simulink model "sampleModel1681_sub"  (R2023a)
settings: Solver=VariableStepAuto  StartTime=0.0  StopTime=10.0  RelTol=1e-3
libraries: hdlsllib x4, simulink x2
settings Model: Creator=user1  LastModifiedBy=user1

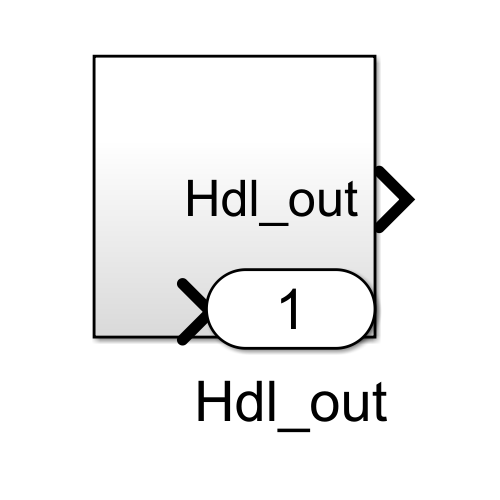
[thumbnail: Simulink's stored preview of the top-level diagram]
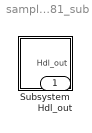
== system sampleModel1681_sub ==
  Subsystem : Subsystem
  Hdl_out : Outport  OutDataTypeStr=uint8

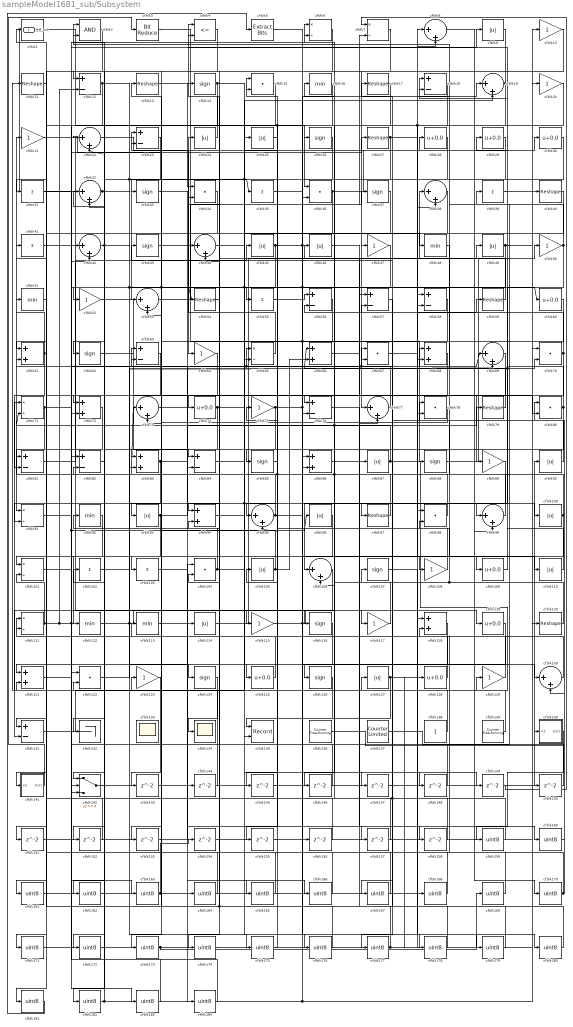
== system sampleModel1681_sub/Subsystem ==
  cfblk1 : simulink/Logic and Bit Operations/Bit Set  iBit=0
      settings: LibrarySourceBlock=|
      | hdlsllib/Logic and Bit
      | Operations/Bit Set
  cfblk{10,20..21,47,50,52,64,75,89,108,115,117,123,129} (14 alike) : Gain  OutDataTypeStr=uint8
  cfblk{9,24..25,45..46,49,87,90,93,96,100,105,110,114,127} (15 alike) : Abs  OutDataTypeStr=uint8  SaturateOnIntegerOverflow=off
  cfblk{6..7,65,71,91,101,111} (7 alike) : Product  Inputs=*/  OutDataTypeStr=uint8  RndMeth=Zero  SaturateOnIntegerOverflow=on
  cfblk{31,35,39,41,55,102..103} (7 alike) : Sum  Inputs=+  OutDataTypeStr=uint8
  cfblk{15,34,36,67,70,78,80,98,104,122} (10 alike) : DotProduct  OutDataTypeStr=uint8
  cfblk{8,19,22,32,38,42,44,53,69,73,77,95,99,106,130} (15 alike) : Sum  Inputs=|++  OutDataTypeStr=uint8
  cfblk{14,26,33,37,43,62,85,88,107,116,124,126} (12 alike) : Signum
  cfblk{28..30,60,74,109,119,125,128} (9 alike) : Bias  Bias=0.0  SaturateOnIntegerOverflow=off
  cfblk{11,13,17,27,40,54,59,79,97,120} (10 alike) : Reshape
  cfblk{16,48,51,92,112..113} (6 alike) : MinMax  OutDataTypeStr=uint8
  cfblk{61,66,68,72,83,86,94,118,121} (9 alike) : Sum  OutDataTypeStr=uint8
  cfblk{12,18,23,56..58,63,76,81..82,84,131} (12 alike) : Sum  Inputs=+-  OutDataTypeStr=uint8
  cfblk132 : Terminator
  cfblk133 : Scope
      settings: Floating=on
  cfblk134 : Scope
  cfblk135 : Record  FileSettingsInternal="{\"entries\":[{\"content\":{\"excelSettings\":{\"content\":{},\"type\":\"Streamout.ExcelSettings\"}},\"type\":\"Streamout.FileSettingStorage\",\"uuid\":\"\"}],\"packageUris\":[\"http:\\/\\/schema.mathworks.com\\/mf0\\/streamout_blocks\\/R2020a\"],\"version\":\"1.0\"}"  Layout=[1 1]  SignalsInternal="{\"entries\":[{\"content\":{\"signals\":[{\"content\":{\"blockPath\":[],\"dimensions\":[1],\"domain\":\"\",\"lineColor\":\"#a2142f\",\"plots\":[1],\"port\":1,\"signalID\":34646,\"signalName\":\"cfblk126\"},\"type\":\"RecordBlkView.Signal\",\"uuid\":\"\"},{\"content\":{\"blockPath\":[],\"dimensions\":[1],\"domain\":\"\",\"lineColor\":\"#139fff\",\"plots\":[1],\"port\":2,\"signalID\":34649,\"signalName\":\"cfblk47\"},\"type\":\"RecordBlkView.Signal\",\"uuid\":\"\"}]},\"type\":\"RecordBlkView.InputSignals\",\"uuid\":\"\"}],\"packageUris\":[\"http:\\/\\/schema.mathworks.com\\/mf0\\/streamout_blocks\\/R2020a\"],\"version\":\"1.0\"}"  VisualizationBindings="{\"xyplotplugin\":{\"info\":[{\"series\":[{\"bindingParametersList\":[{\"parameter\":\"X-Axis\",\"signalID\":34646,\"signalName\":\"cfblk126\"},{\"parameter\":\"Y-Axis\",\"signalID\":34649,\"signalName\":\"cfblk47\"}],\"seriesID\":4685}],\"subplotID\":1}]}}"  CompatibilityTag=XY  st=-1
  cfblk136 : hdlsllib/Sources/Counter Free-Running  NumBits=16  tsamp=-1
  cfblk137 : hdlsllib/Sources/Counter Limited  uplimit=7  tsamp=-1
  cfblk138 : Constant  OutDataTypeStr=uint8  SampleTime=-1
  cfblk139 : hdlsllib/Sources/Counter Free-Running  NumBits=16  tsamp=-1
  cfblk140 : Subsystem
      settings: LibrarySourceBlock=|
      | hdlsllib/Ports &
      | Subsystems/Subsystem
  cfblk141 : Subsystem
      settings: LibrarySourceBlock=|
      | hdlsllib/Ports &
      | Subsystems/Subsystem
  cfblk142 : Switch  OutDataTypeStr=uint8  SaturateOnIntegerOverflow=off  InputSameDT=off
  cfblk{143..158} (16 alike) : Delay  SampleTime=1
  cfblk{159..184} (26 alike) : DataTypeConversion  OutDataTypeStr=uint8  SaturateOnIntegerOverflow=off  RndMeth=Floor
  cfblk2 : Logic  AllPortsSameDT=off  OutDataTypeStr=boolean
  cfblk3 : hdlsllib/Logic and Bit Operations/Bit Reduce  mode=AND
  cfblk4 : RelationalOperator  Operator=<=  OutDataTypeStr=boolean  InputSameDT=off
  cfblk5 : simulink/Logic and Bit Operations/Extract Bits  bitsToExtract=Upper half  numBits=8  bitIdxRange=[0 7]  outScalingMode=Preserve fixed-point scaling
      settings: LibrarySourceBlock=|
      | hdlsllib/Logic and Bit
      | Operations/Extract Bits
  Hdl_out : Outport  OutDataTypeStr=uint8
  wires:
  cfblk21/1 -> cfblk119/1
  cfblk52/1 -> cfblk84/1
  cfblk93/1 -> cfblk79/1, cfblk112/1
  cfblk125/1 -> cfblk111/1
  cfblk138/1 -> cfblk11/1
  cfblk63/1 -> cfblk142/1
  cfblk24/1 -> cfblk4/1
  cfblk119/1 -> cfblk121/1
  cfblk87/1 -> cfblk44/1, cfblk129/1
  cfblk7/1 -> cfblk77/1
  cfblk78/1 -> cfblk22/1
  cfblk61/1 -> cfblk81/2, cfblk21/1
  cfblk77/1 -> cfblk2/2, cfblk67/1
  cfblk137/1 -> cfblk39/1
  cfblk22/1 -> cfblk64/1
  cfblk88/1 -> cfblk50/1
  cfblk26/1 -> cfblk162/1, cfblk65/2
  cfblk2/1 -> cfblk31/1
  cfblk97/1 -> cfblk75/1, cfblk73/1
  cfblk36/1 -> cfblk141/1(In1), cfblk30/1
  cfblk141/1(Out1) -> cfblk3/1
  cfblk81/1 -> cfblk45/1
  cfblk29/1 -> cfblk47/1
  cfblk3/1 -> cfblk88/1
  cfblk1/1 -> cfblk36/1
  cfblk51/1 -> cfblk91/1
  cfblk99/1 -> cfblk78/1
  cfblk114/1 -> cfblk38/1
  cfblk84/1 -> cfblk178/1, cfblk99/2
  cfblk4/1 -> cfblk62/1
  cfblk10/1 -> cfblk173/1
  cfblk39/1 -> cfblk20/1
  cfblk98/1 -> cfblk56/2, cfblk32/1
  cfblk111/1 -> cfblk101/2, cfblk12/2, cfblk183/1, cfblk65/1, cfblk69/1
  cfblk70/1 -> cfblk6/2, cfblk93/1
  cfblk75/1 -> cfblk94/1, cfblk19/1, cfblk109/1
  cfblk65/1 -> cfblk24/1
  cfblk126/1 -> cfblk135/1
  cfblk139/1 -> cfblk46/1
  cfblk100/1 -> cfblk106/2, cfblk51/1
  cfblk66/1 -> cfblk49/1
  cfblk20/1 -> cfblk68/2, cfblk86/2
  cfblk105/1 -> cfblk66/2, cfblk73/2
  cfblk59/1 -> cfblk14/1
  cfblk108/1 -> cfblk23/1
  cfblk57/1 -> cfblk177/1
  cfblk109/1 -> cfblk29/1
  cfblk64/1 -> cfblk131/1
  cfblk58/1 -> cfblk97/1
  cfblk47/1 -> cfblk135/2, cfblk84/2
  cfblk12/1 -> cfblk142/2, cfblk35/1, cfblk54/1, cfblk100/1
  cfblk106/1 -> cfblk131/2
  cfblk23/1 -> cfblk72/1
  cfblk55/1 -> cfblk56/1
  cfblk45/1 -> cfblk37/1, cfblk130/1, cfblk60/1, cfblk103/1, cfblk83/2
  cfblk131/1 -> cfblk25/1
  cfblk89/1 -> cfblk106/1
  cfblk41/1 -> cfblk163/1
  cfblk13/1 -> cfblk34/1
  cfblk18/1 -> cfblk95/2, cfblk61/1
  cfblk127/1 -> cfblk179/1, cfblk155/1
  cfblk27/1 -> cfblk110/1, cfblk53/1
  cfblk83/1 -> cfblk91/2, cfblk68/1
  cfblk68/1 -> cfblk126/1
  cfblk115/1 -> cfblk160/1, cfblk117/1
  cfblk122/1 -> cfblk70/2
  cfblk6/1 -> cfblk52/1
  cfblk30/1 -> cfblk116/1
  cfblk43/1 -> cfblk114/1
  cfblk129/1 -> cfblk94/2
  cfblk136/1 -> cfblk80/1
  cfblk71/1 -> cfblk81/1, cfblk27/1
  cfblk28/1 -> cfblk85/1
  cfblk95/1 -> cfblk147/1, cfblk44/2
  cfblk110/1 -> cfblk18/2, cfblk66/1
  cfblk11/1 -> cfblk101/1
  cfblk112/1 -> cfblk69/2, cfblk115/1
  cfblk116/1 -> cfblk125/1
  cfblk82/1 -> cfblk182/1
  cfblk17/1 -> cfblk26/1
  cfblk56/1 -> cfblk95/1
  cfblk67/1 -> cfblk59/1
  cfblk50/1 -> cfblk99/1, cfblk2/1
  cfblk104/1 -> cfblk166/1, cfblk32/2
  cfblk76/1 -> cfblk87/1
  cfblk42/1 -> cfblk176/1, cfblk22/2
  cfblk101/1 -> cfblk42/1
  cfblk15/1 -> cfblk142/3
  cfblk62/1 -> cfblk98/1
  cfblk80/1 -> cfblk172/1, cfblk4/2
  cfblk16/1 -> cfblk33/1
  cfblk140/1(Out1) -> cfblk159/1
  cfblk130/1 -> cfblk107/1
  cfblk69/1 -> cfblk89/1
  cfblk74/1 -> cfblk152/1, cfblk19/2
  cfblk5/1 -> cfblk180/1
  cfblk90/1 -> cfblk43/1
  cfblk121/1 -> cfblk9/1, cfblk96/1
  cfblk79/1 -> cfblk18/1
  cfblk142/1 -> cfblk90/1
  cfblk94/1 -> cfblk28/1
  cfblk128/1 -> cfblk15/1
  cfblk91/1 -> cfblk42/2
  cfblk32/1 -> Hdl_out/1, cfblk58/2, cfblk124/1
  cfblk53/1 -> cfblk7/2
  cfblk120/1 -> cfblk98/2, cfblk61/2
  cfblk9/1 -> cfblk74/1
  cfblk19/1 -> cfblk12/1, cfblk76/1
  cfblk40/1 -> cfblk78/2
  cfblk49/1 -> cfblk72/2, cfblk40/1
  cfblk8/1 -> cfblk170/1
  cfblk46/1 -> cfblk80/2
  cfblk96/1 -> cfblk132/1
  cfblk48/1 -> cfblk108/1
  cfblk31/1 -> cfblk6/1
  cfblk124/1 -> cfblk134/1
  cfblk117/1 -> cfblk63/1, cfblk71/2
  cfblk14/1 -> cfblk153/1, cfblk48/1
  cfblk60/1 -> cfblk83/1, cfblk76/2
  cfblk25/1 -> cfblk55/1
  cfblk123/1 -> cfblk143/1
  cfblk73/1 -> cfblk144/1
  cfblk144/1 -> cfblk71/1
  cfblk85/1 -> cfblk145/1
  cfblk145/1 -> cfblk77/2
  cfblk38/1 -> cfblk146/1
  cfblk146/1 -> cfblk23/2
  cfblk147/1 -> cfblk67/2
  cfblk44/1 -> cfblk148/1
  cfblk148/1 -> cfblk58/1
  cfblk35/1 -> cfblk149/1
  cfblk149/1 -> cfblk7/1
  cfblk150/1 -> cfblk122/1
  cfblk34/1 -> cfblk151/1
  cfblk151/1 -> cfblk104/1
  cfblk152/1 -> cfblk111/2
  cfblk153/1 -> cfblk53/2
  cfblk154/1 -> cfblk36/2
  cfblk155/1 -> cfblk70/1
  cfblk156/1 -> cfblk1/1
  cfblk33/1 -> cfblk157/1
  cfblk157/1 -> cfblk16/1
  cfblk86/1 -> cfblk158/1
  cfblk158/1 -> cfblk17/1
  cfblk159/1 -> cfblk127/1, cfblk105/1
  cfblk160/1 -> cfblk140/1(In1)
  cfblk92/1 -> cfblk161/1
  cfblk161/1 -> cfblk86/1
  cfblk162/1 -> cfblk92/1
  cfblk163/1 -> cfblk38/2, cfblk154/1
  cfblk103/1 -> cfblk164/1
  cfblk164/1 -> cfblk41/1
  cfblk113/1 -> cfblk165/1
  cfblk165/1 -> cfblk123/1
  cfblk166/1 -> cfblk113/1
  cfblk118/1 -> cfblk167/1
  cfblk167/1 -> cfblk13/1
  cfblk107/1 -> cfblk168/1
  cfblk168/1 -> cfblk118/1
  cfblk169/1 -> cfblk118/2
  cfblk170/1 -> cfblk34/2, cfblk130/2
  cfblk37/1 -> cfblk171/1
  cfblk171/1 -> cfblk8/1
  cfblk172/1 -> cfblk8/2
  cfblk173/1 -> cfblk150/1, cfblk169/1
  cfblk54/1 -> cfblk174/1
  cfblk174/1 -> cfblk10/1
  cfblk102/1 -> cfblk175/1
  cfblk175/1 -> cfblk15/2
  cfblk176/1 -> cfblk102/1
  cfblk177/1 -> cfblk128/1, cfblk63/2
  cfblk178/1 -> cfblk57/1
  cfblk179/1 -> cfblk57/2
  cfblk180/1 -> cfblk104/2, cfblk121/2
  cfblk72/1 -> cfblk181/1
  cfblk181/1 -> cfblk5/1
  cfblk182/1 -> cfblk122/2, cfblk120/1, cfblk156/1
  cfblk183/1 -> cfblk82/1
  cfblk143/1 -> cfblk184/1
  cfblk184/1 -> cfblk82/2

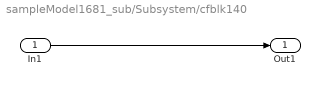
== system sampleModel1681_sub/Subsystem/cfblk140 ==
  In1 : Inport
  Out1 : Outport
  wires:
  In1/1 -> Out1/1

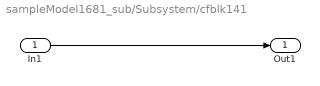
== system sampleModel1681_sub/Subsystem/cfblk141 ==
  In1 : Inport
  Out1 : Outport
  wires:
  In1/1 -> Out1/1
